simulink model "Vehicle1DBasic_test_harness"  (R2020b)
settings: Solver=ode23t  StartTime=0.0  StopTime=t_end  RelTol=1e-3  AbsTol=1e-3
PreLoadFcn:
  | Vehicle1DBasic_setup
undefined symbols (not defined in the file or in its folder): gearTrain
libraries: fl_lib x5, nesl_utility x2
settings Model: Creator=isaacito  LastModifiedBy=isaacito
settings SolverCC: AutoScaleAbsTol=off
settings SimscapeCC: SimscapeLogType=all  SimscapeLogSimulationStatistics=on  SimscapeLogLimitData=off

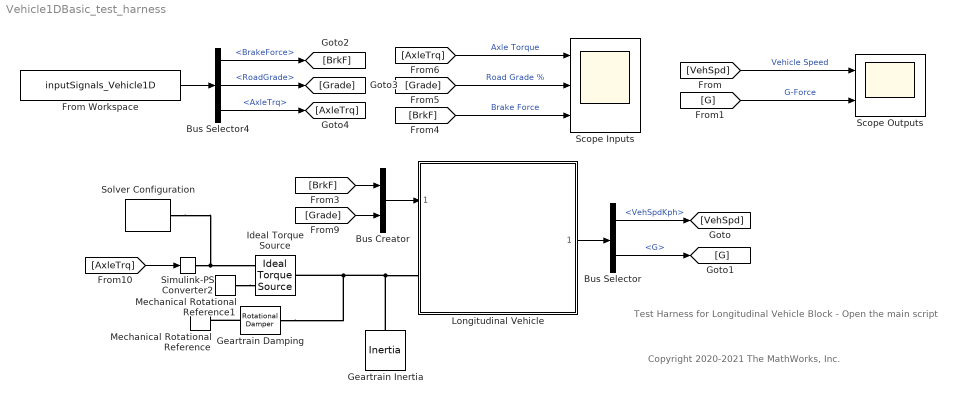
== system Vehicle1DBasic_test_harness ==
  note: Test Harness for Longitudinal Vehicle Block
      | - Open the main script
  note: Copyright 2020-2021 The MathWorks, Inc.
  Bus Creator : BusCreator  Inputs=2
  Bus Selector : BusSelector  OutputSignals=VehSpdKph,G
  Bus Selector4 : BusSelector  OutputSignals=BrakeForce,RoadGrade,AxleTrq
  From Workspace : FromWorkspace  VariableName=inputSignals_Vehicle1D  OutDataTypeStr=Bus: inputBus_Vehicle1D  Interpolate=off  OutputAfterFinalValue=Holding final value
      settings: AttributesFormatString=|
      | %<OutDataTypeStr>
      | Interpolate: %<Interpolate>
  Geartrain Damping : fl_lib/Mechanical/Rotational Elements/Rotational Damper  D=gearTrain.friction_Nm_per_rpm m*N/rpm  w_specify=off  w_priority=None  w=0 rad/s  w_nominal_specify=off  w_nominal_unit=rad/s  w_nominal_value=1  t_specify=off  t_priority=None  t=0 N*m  t_nominal_specify=off  t_nominal_unit=N*m  t_nominal_value=1
      settings: AttributesFormatString=|
      | %<D>
      | %<D_unit>
  Geartrain Inertia : fl_lib/Mechanical/Rotational Elements/Inertia  inertia=gearTrain.inertia_kg_m2 kg*m^2  num_ports=foundation.enum.numPorts2.one  w_specify=on  w_priority=High  w=initial.GeartrainSpeed_rpm rpm  w_nominal_specify=off  w_nominal_unit=rad/s  w_nominal_value=1  t_specify=off  t_priority=None  t=0 N*m  t_nominal_specify=off  t_nominal_unit=N*m  t_nominal_value=1
      settings: AttributesFormatString=|
      | %<inertia>
      | %<inertia_unit>
  Ideal Torque Source : fl_lib/Mechanical/Mechanical Sources/Ideal Torque Source
  Longitudinal Vehicle : Subsystem  ReferencedSubsystem=Vehicle1DBasic_refsub
  Mechanical Rotational Reference : fl_lib/Mechanical/Rotational Elements/Mechanical Rotational Reference
  Mechanical Rotational Reference1 : fl_lib/Mechanical/Rotational Elements/Mechanical Rotational Reference
  Scope Inputs : Scope  NumInputPorts=3
  Scope Outputs : Scope  NumInputPorts=2
  Simulink-PS Converter2 : nesl_utility/Simulink-PS Converter  PhysicalDomain=network_engine_domain  SubClassName=ps_input  LeftPortType=input  RightPortType=output  PseudoPeriodic=off  Frequencies=[]  NoiseDistribution=none  NoiseParameters=[]  Unit=N*m  AffineConversion=off  FilteringAndDerivatives=provide  SimscapeFilterOrder=1  InputFilterTimeConstant=0.001  UdotUserProvided=0
  Solver Configuration : nesl_utility/Solver Configuration  PhysicalDomain=network_engine_domain  SubClassName=solver  LeftPortType=input  RightPortType=generic  Tones=[]  Harmonics=[]  SimulateNoise=off  Profile=off  UseLocalSampling=off  EnableSwitchedLinearOptims=on  FrequencyDomain=off  UseCCode=off  RelTol=0.001  AbsTol=1e-06  MinStep=1e-09  ToWorkspace=off  RevertToSquareIcSolve=off  NumHomotopyIterations=100  PhasorMode=off  PhasorModeNumHarmonics=1  DoDC=off  ResidualTolerance=1e-09  UseLocalSolver=off  LocalSolverChoice=NE_BACKWARD_EULER_ADVANCER  LocalSolverSampleTime=0.001  DoFixedCost=off  MaxNonlinIter=3  MaxModeIter=2  ComputeImpulses=off  ImpulseIterations=2  LinearAlgebra=auto  EquationFormulation=NE_TIME_EF  DelaysMemoryBudget=1024  AutomaticFiltering=on  FilteringTimeConstant=0.001  PartitionStorageMethod=AS_NEEDED  PartitionMemoryBudget=1024  PartitionMethod=ROBUST
      settings: AttributesFormatString=Local solver %<UseLocalSolver>
  wires:
  [G] -> Scope Outputs/2  "G-Force"
  [VehSpd] -> Scope Outputs/1  "Vehicle Speed"
  Bus Selector/1 -> [VehSpd]  "<VehSpdKph>"
  Bus Selector/2 -> [G]  "<G>"
  Longitudinal Vehicle/1 -> Bus Selector/1
  Bus Creator/1 -> Longitudinal Vehicle/1
  [Grade] -> Scope Inputs/2  "Road Grade %"
  [BrkF] -> Scope Inputs/3  "Brake Force"
  [AxleTrq] -> Scope Inputs/1  "Axle Torque"
  [BrkF] -> Bus Creator/1
  [Grade] -> Bus Creator/2
  [AxleTrq] -> Simulink-PS Converter2/1
  From Workspace/1 -> Bus Selector4/1
  Bus Selector4/1 -> [BrkF]  "<BrakeForce>"
  Bus Selector4/2 -> [Grade]  "<RoadGrade>"
  Bus Selector4/3 -> [AxleTrq]  "<AxleTrq>"
  connections:
  Geartrain Damping/RConn1 -- Mechanical Rotational Reference/LConn1
  Simulink-PS Converter2/RConn1 -- Ideal Torque Source/RConn1 -- Solver Configuration/RConn1
  Geartrain Inertia/LConn1 -- Ideal Torque Source/LConn1 -- Geartrain Damping/LConn1 -- Longitudinal Vehicle/LConn1
  Mechanical Rotational Reference1/LConn1 -- Ideal Torque Source/RConn2
